simulink model "Part1_NDP_InfiniteBuffer"  (R2024b)
settings: Solver=ode45  StartTime=0.0  StopTime=10  MaxStep=0.01  RelTol=1e-3
settings Model: Creator=SherOu  LastModifiedBy=SherOu

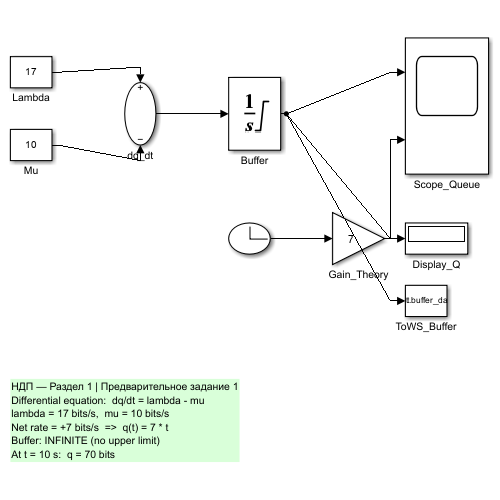
[thumbnail: Simulink's stored preview of the top-level diagram]
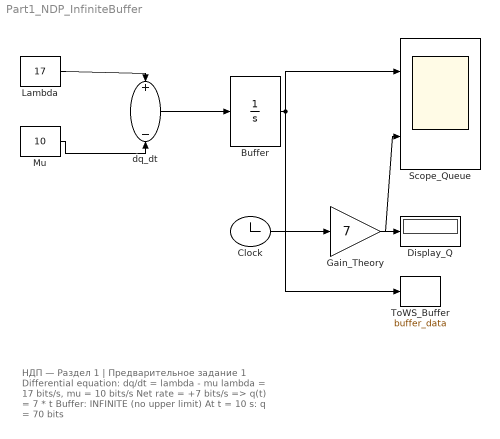
== system Part1_NDP_InfiniteBuffer ==
  note: НДП — Раздел 1 | Предварительное задание 1
      | Differential equation:  dq/dt = lambda - mu
      | lambda = 17 bits/s,  mu = 10 bits/s
      | Net rate = +7 bits/s  =>  q(t) = 7 * t
      | Buffer: INFINITE (no upper limit)
      | At t = 10 s:  q = 70 bits
  Buffer : Integrator  LimitOutput=on  LowerSaturationLimit=0
  Clock : Clock
  Display_Q : Display
  Gain_Theory : Gain  Gain=7
  Lambda : Constant  Value=17
  Mu : Constant  Value=10
  Scope_Queue : Scope  NumInputPorts=2
  ToWS_Buffer : ToWorkspace  VariableName=buffer_data  SampleTime=-1
  dq_dt : Sum  Inputs=+-
  wires:
  Lambda/1 -> dq_dt/1
  Mu/1 -> dq_dt/2
  dq_dt/1 -> Buffer/1
  Buffer/1 -> Scope_Queue/1, Display_Q/1, ToWS_Buffer/1
  Clock/1 -> Gain_Theory/1
  Gain_Theory/1 -> Scope_Queue/2
